simulink model "Projekt_ABS_Sim_Fuzzy"  (R2024b)
settings: Solver=VariableStepAuto  StartTime=0.0  StopTime=10  RelTol=1e-3
values from neighbouring files (symbols this model uses):
  c1 = 0.857    [Projekt_ABS.m]
  c11 = 1.2801    [Projekt_ABS.m]
  c2 = 33.822    [Projekt_ABS.m]
  c22 = 23.99    [Projekt_ABS.m]
  c3 = 0.347    [Projekt_ABS.m]
  c33 = 0.52    [Projekt_ABS.m]
  c4 = 0.035    [Projekt_ABS.m]
  c44 = 0.03    [Projekt_ABS.m]
  g = 9.81    [Projekt_ABS.m]
  J = 1.6    [Projekt_ABS.m]
  m = 1200    [Projekt_ABS.m]
  Mb = 900    [Projekt_ABS.m]
  R = 0.315    [Projekt_ABS.m]
  Ts = 0.01    [Projekt_ABS.m]
  V0 = 40    [Projekt_ABS.m]
undefined symbols (not defined in the file or in its folder): DiscIntNeverNeededParam
libraries: fuzblock x6, simulink x4
settings Model: Creator=abc  LastModifiedBy=abc

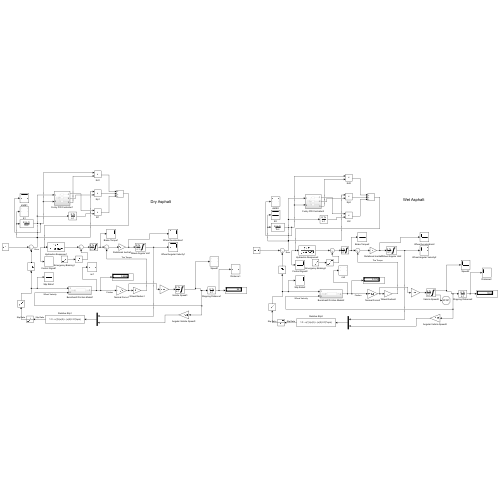
[thumbnail: Simulink's stored preview of the top-level diagram]
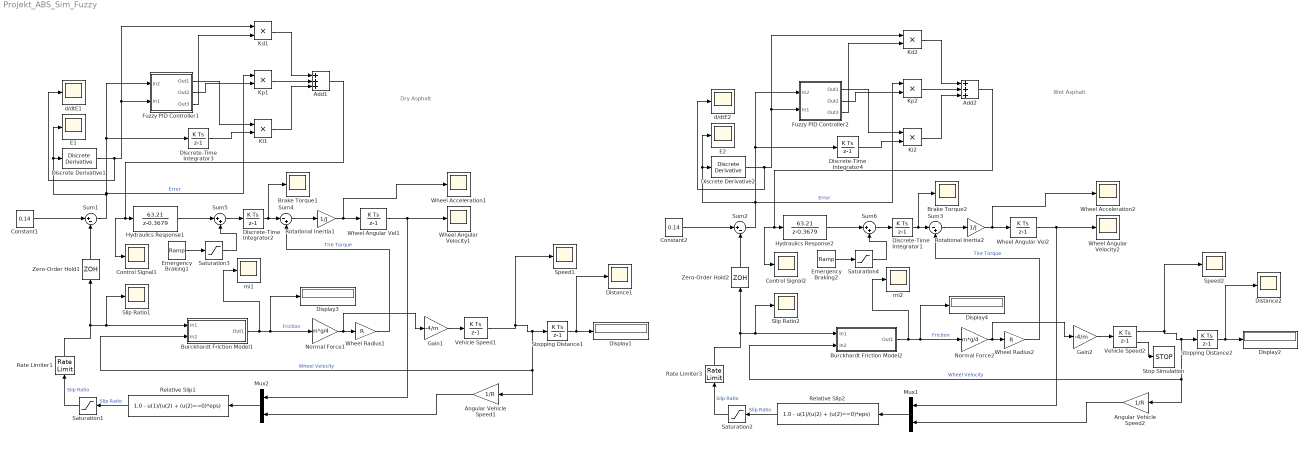
== system Projekt_ABS_Sim_Fuzzy ==
  note: Dry Asphalt
  note: Wet Asphalt
  Add1 : Sum  Inputs=+++
  Add2 : Sum  Inputs=+++
  Angular Vehicle Speed1 : Gain  Gain=1/R
  Angular Vehicle Speed2 : Gain  Gain=1/R
  Brake Torque1 : Scope
  Brake Torque2 : Scope
  Burckhardt Friction Model1 : Subsystem
  Burckhardt Friction Model2 : Subsystem
  Constant1 : Constant  Value=0.14  SampleTime=Ts
  Constant2 : Constant  Value=0.14  SampleTime=Ts
  Control Signal1 : Scope
  Control Signal2 : Scope
  Discrete Derivative1 : simulink/Quick Insert/Discrete/Discrete Derivative  gainval=1.0  ICPrevScaledInput=0.0  OutMin=[]  OutMax=[]  OutDataType=fixdt(1, 16)  OutScaling=2^-10  DoSatur=off
  Discrete Derivative2 : simulink/Quick Insert/Discrete/Discrete Derivative  gainval=1.0  ICPrevScaledInput=0.0  OutMin=[]  OutMax=[]  OutDataType=fixdt(1, 16)  OutScaling=2^-10  DoSatur=off
  Discrete-Time Integrator1 : DiscreteIntegrator  SampleTime=Ts  LimitOutput=on  UpperSaturationLimit=Mb  LowerSaturationLimit=0  ICPrevOutput=DiscIntNeverNeededParam  ICPrevScaledInput=DiscIntNeverNeededParam
  Discrete-Time Integrator2 : DiscreteIntegrator  SampleTime=Ts  LimitOutput=on  UpperSaturationLimit=Mb  LowerSaturationLimit=0  ICPrevOutput=DiscIntNeverNeededParam  ICPrevScaledInput=DiscIntNeverNeededParam
  Discrete-Time Integrator3 : DiscreteIntegrator  SampleTime=Ts  ICPrevOutput=DiscIntNeverNeededParam  ICPrevScaledInput=DiscIntNeverNeededParam
  Discrete-Time Integrator4 : DiscreteIntegrator  SampleTime=Ts  ICPrevOutput=DiscIntNeverNeededParam  ICPrevScaledInput=DiscIntNeverNeededParam
  Display{1..4} (4 alike) : Display
  Distance1 : Scope
  Distance2 : Scope
  E1 : Scope
  E2 : Scope
  Emergency Braking1 : simulink/Sources/Ramp  slope=Mb*2  start=0  InitialOutput=0
  Emergency Braking2 : simulink/Sources/Ramp  slope=Mb*2  start=0  InitialOutput=0
  Fuzzy PID Controller1 : Subsystem
  Fuzzy PID Controller2 : Subsystem
  Gain1 : Gain  Gain=-4/m
  Gain2 : Gain  Gain=-4/m
  Hydraulics Response1 : DiscreteTransferFcn  Numerator=[63.21]  Denominator=[1 -0.3679]  SampleTime=Ts
  Hydraulics Response2 : DiscreteTransferFcn  Numerator=[63.21]  Denominator=[1 -0.3679]  SampleTime=Ts
  Kd1 : Product
  Kd2 : Product
  Ki1 : Product
  Ki2 : Product
  Kp1 : Product
  Kp2 : Product
  Mux1 : Mux  Inputs=2
  Mux2 : Mux  Inputs=2
  Normal Force1 : Gain  Gain=m*g/4
  Normal Force2 : Gain  Gain=m*g/4
  Rate Limiter1 : RateLimiter  RisingSlewLimit=1.5  FallingSlewLimit=-1.5  SampleTimeMode=inherited
  Rate Limiter3 : RateLimiter  RisingSlewLimit=1.5  FallingSlewLimit=-1.5  SampleTimeMode=inherited
  Relative Slip1 : Fcn  Expr=1.0 - u(1)/(u(2) + (u(2)==0)*eps)
  Relative Slip2 : Fcn  Expr=1.0 - u(1)/(u(2) + (u(2)==0)*eps)
  Rotational Inertia1 : Gain  Gain=1/J
  Rotational Inertia2 : Gain  Gain=1/J
  Saturation1 : Saturate  UpperLimit=1  LowerLimit=0
  Saturation2 : Saturate  UpperLimit=1  LowerLimit=0
  Saturation3 : Saturate  UpperLimit=Mb  LowerLimit=0
  Saturation4 : Saturate  UpperLimit=Mb  LowerLimit=0
  Slip Ratio1 : Scope
  Slip Ratio2 : Scope
  Speed1 : Scope
  Speed2 : Scope
  Stop Simulation : Stop
  Stopping Distance1 : DiscreteIntegrator  SampleTime=Ts  ICPrevOutput=DiscIntNeverNeededParam  ICPrevScaledInput=DiscIntNeverNeededParam
  Stopping Distance2 : DiscreteIntegrator  SampleTime=Ts  ICPrevOutput=DiscIntNeverNeededParam  ICPrevScaledInput=DiscIntNeverNeededParam
  Sum1 : Sum  Inputs=|+-
  Sum2 : Sum  Inputs=|+-
  Sum3 : Sum  Inputs=|-+
  Sum4 : Sum  Inputs=|-+
  Sum5 : Sum  Inputs=|++
  Sum6 : Sum  Inputs=|++
  Vehicle Speed1 : DiscreteIntegrator  InitialCondition=V0  SampleTime=Ts  LimitOutput=on  UpperSaturationLimit=1000  LowerSaturationLimit=0  ICPrevOutput=DiscIntNeverNeededParam  ICPrevScaledInput=DiscIntNeverNeededParam
  Vehicle Speed2 : DiscreteIntegrator  InitialCondition=V0  SampleTime=Ts  LimitOutput=on  UpperSaturationLimit=1000  LowerSaturationLimit=0  ShowSaturationPort=on  ICPrevOutput=DiscIntNeverNeededParam  ICPrevScaledInput=DiscIntNeverNeededParam
  Wheel Acceleration1 : Scope
  Wheel Acceleration2 : Scope
  Wheel Angular Vel1 : DiscreteIntegrator  InitialCondition=V0/R  SampleTime=Ts  LimitOutput=on  UpperSaturationLimit=1000  LowerSaturationLimit=0  ICPrevOutput=DiscIntNeverNeededParam  ICPrevScaledInput=DiscIntNeverNeededParam
  Wheel Angular Vel2 : DiscreteIntegrator  InitialCondition=V0/R  SampleTime=Ts  LimitOutput=on  UpperSaturationLimit=1000  LowerSaturationLimit=0  ICPrevOutput=DiscIntNeverNeededParam  ICPrevScaledInput=DiscIntNeverNeededParam
  Wheel Angular Velocity1 : Scope
  Wheel Angular Velocity2 : Scope
  Wheel Radius1 : Gain  Gain=R
  Wheel Radius2 : Gain  Gain=R
  Zero-Order Hold1 : ZeroOrderHold  SampleTime=Ts
  Zero-Order Hold2 : ZeroOrderHold  SampleTime=Ts
  d/dtE1 : Scope
  d/dtE2 : Scope
  mi1 : Scope
  mi2 : Scope
  wires:
  Normal Force1/1 -> Gain1/1, Wheel Radius1/1
  Kp1/1 -> Add1/2
  Sum1/1 -> Kp1/1, Discrete-Time Integrator3/1, Fuzzy PID Controller1/1(In2), Discrete Derivative1/1, E1/1  "Error"
  Zero-Order Hold1/1 -> Sum1/2
  Discrete-Time Integrator2/1 -> Brake Torque1/1, Sum4/1
  Wheel Angular Vel1/1 -> Wheel Angular Velocity1/1, Mux2/1
  Ki1/1 -> Add1/3
  Add1/1 -> Control Signal1/1, Hydraulics Response1/1
  Kd1/1 -> Add1/1
  Discrete Derivative1/1 -> d/dtE1/1, Kd1/1, Fuzzy PID Controller1/2(In1)
  Discrete-Time Integrator3/1 -> Ki1/2
  Fuzzy PID Controller1/1(Out1) -> Ki1/1
  Relative Slip1/1 -> Saturation1/1  "Slip Ratio"
  Saturation1/1 -> Rate Limiter1/1  "Slip Ratio"
  Wheel Radius1/1 -> Sum4/2  "Tire Torque"
  Vehicle Speed1/1 -> Speed1/1, Stopping Distance1/1, Burckhardt Friction Model1/2(In2), Angular Vehicle Speed1/1  "Wheel Velocity"
  Stopping Distance1/1 -> Distance1/1, Display1/1
  Fuzzy PID Controller1/2(Out2) -> Kp1/2
  Burckhardt Friction Model1/1(Out1) -> mi1/1, Display3/1, Normal Force1/1  "Friction"
  Mux2/1 -> Relative Slip1/1
  Rotational Inertia1/1 -> Wheel Angular Vel1/1, Wheel Acceleration1/1
  Rate Limiter1/1 -> Zero-Order Hold1/1, Slip Ratio1/1, Burckhardt Friction Model1/1(In1)
  Gain1/1 -> Vehicle Speed1/1
  Fuzzy PID Controller1/3(Out3) -> Kd1/2
  Sum4/1 -> Rotational Inertia1/1
  Angular Vehicle Speed1/1 -> Mux2/2
  Constant1/1 -> Sum1/1
  Emergency Braking1/1 -> Saturation3/1
  Saturation3/1 -> Sum5/2
  Hydraulics Response1/1 -> Sum5/1
  Sum5/1 -> Discrete-Time Integrator2/1
  Discrete Derivative2/1 -> d/dtE2/1, Kd2/1, Fuzzy PID Controller2/2(In1)
  Gain2/1 -> Vehicle Speed2/1
  Kd2/1 -> Add2/1
  Vehicle Speed2/1 -> Stopping Distance2/1, Burckhardt Friction Model2/2(In2), Angular Vehicle Speed2/1, Speed2/1  "Wheel Velocity"
  Ki2/1 -> Add2/3
  Hydraulics Response2/1 -> Sum6/1
  Wheel Angular Vel2/1 -> Wheel Angular Velocity2/1, Mux1/1
  Fuzzy PID Controller2/1(Out1) -> Ki2/1
  Saturation2/1 -> Rate Limiter3/1  "Slip Ratio"
  Rate Limiter3/1 -> Zero-Order Hold2/1, Slip Ratio2/1, Burckhardt Friction Model2/1(In1)
  Kp2/1 -> Add2/2
  Normal Force2/1 -> Gain2/1, Wheel Radius2/1
  Emergency Braking2/1 -> Saturation4/1
  Zero-Order Hold2/1 -> Sum2/2
  Burckhardt Friction Model2/1(Out1) -> mi2/1, Display4/1, Normal Force2/1  "Friction"
  Mux1/1 -> Relative Slip2/1
  Saturation4/1 -> Sum6/2
  Fuzzy PID Controller2/2(Out2) -> Kp2/2
  Sum3/1 -> Rotational Inertia2/1
  Wheel Radius2/1 -> Sum3/2  "Tire Torque"
  Sum2/1 -> Kp2/1, Discrete-Time Integrator4/1, Fuzzy PID Controller2/1(In2), Discrete Derivative2/1, E2/1  "Error"
  Sum6/1 -> Discrete-Time Integrator1/1
  Stopping Distance2/1 -> Distance2/1, Display2/1
  Angular Vehicle Speed2/1 -> Mux1/2
  Relative Slip2/1 -> Saturation2/1  "Slip Ratio"
  Discrete-Time Integrator1/1 -> Brake Torque2/1, Sum3/1
  Fuzzy PID Controller2/3(Out3) -> Kd2/2
  Discrete-Time Integrator4/1 -> Ki2/2
  Constant2/1 -> Sum2/1
  Add2/1 -> Control Signal2/1, Hydraulics Response2/1
  Rotational Inertia2/1 -> Wheel Angular Vel2/1, Wheel Acceleration2/1
  Vehicle Speed2/2 -> Stop Simulation/1

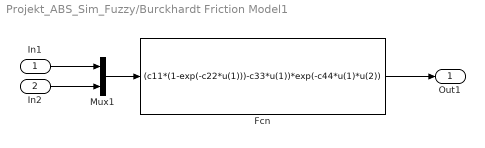
== system Projekt_ABS_Sim_Fuzzy/Burckhardt Friction Model1 ==
  In1 : Inport
  In2 : Inport  Port=2
  Fcn : Fcn  Expr=(c11*(1-exp(-c22*u(1)))-c33*u(1))*exp(-c44*u(1)*u(2))
  Mux1 : Mux  Inputs=2
  Out1 : Outport
  wires:
  In2/1 -> Mux1/2
  Mux1/1 -> Fcn/1
  In1/1 -> Mux1/1
  Fcn/1 -> Out1/1

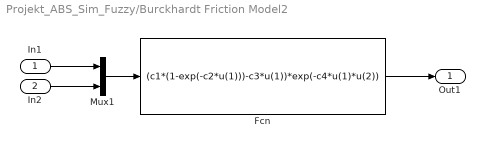
== system Projekt_ABS_Sim_Fuzzy/Burckhardt Friction Model2 ==
  In1 : Inport
  In2 : Inport  Port=2
  Fcn : Fcn  Expr=(c1*(1-exp(-c2*u(1)))-c3*u(1))*exp(-c4*u(1)*u(2))
  Mux1 : Mux  Inputs=2
  Out1 : Outport
  wires:
  In2/1 -> Mux1/2
  Mux1/1 -> Fcn/1
  In1/1 -> Mux1/1
  Fcn/1 -> Out1/1

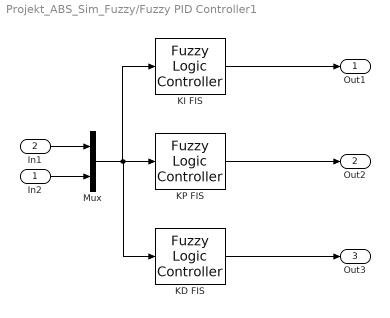
== system Projekt_ABS_Sim_Fuzzy/Fuzzy PID Controller1 ==
  In2 : Inport
  In1 : Inport  Port=2
  KD FIS : fuzblock/Fuzzy Logic  Controller  FIS='KD.fis'  OutputSampleNumber=101  DataType=double  FuzzifiedInputs=off  RuleFiringStrengths=off  RuleOutputs=off  AggregatedOutputs=off  SimulateUsing=Interpreted execution  OutOfRangeInputValueMessage=warning  NoRuleFiredMessage=warning  EmptyOutputFuzzySetMessage=warning
  KI FIS : fuzblock/Fuzzy Logic  Controller  FIS='KI.fis'  OutputSampleNumber=101  DataType=double  FuzzifiedInputs=off  RuleFiringStrengths=off  RuleOutputs=off  AggregatedOutputs=off  SimulateUsing=Interpreted execution  OutOfRangeInputValueMessage=warning  NoRuleFiredMessage=warning  EmptyOutputFuzzySetMessage=warning
  KP FIS : fuzblock/Fuzzy Logic  Controller  FIS='KP.fis'  OutputSampleNumber=101  DataType=double  FuzzifiedInputs=off  RuleFiringStrengths=off  RuleOutputs=off  AggregatedOutputs=off  SimulateUsing=Interpreted execution  OutOfRangeInputValueMessage=warning  NoRuleFiredMessage=warning  EmptyOutputFuzzySetMessage=warning
  Mux : Mux  Inputs=2
  Out1 : Outport
  Out2 : Outport  Port=2
  Out3 : Outport  Port=3
  wires:
  Mux/1 -> KI FIS/1, KD FIS/1, KP FIS/1
  In1/1 -> Mux/1
  KI FIS/1 -> Out1/1
  KD FIS/1 -> Out3/1
  KP FIS/1 -> Out2/1
  In2/1 -> Mux/2

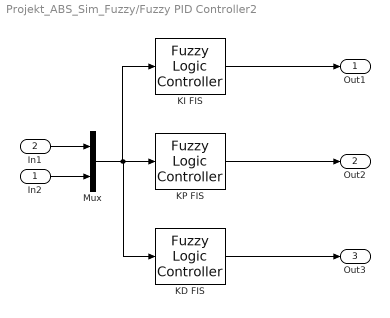
== system Projekt_ABS_Sim_Fuzzy/Fuzzy PID Controller2 ==
  In2 : Inport
  In1 : Inport  Port=2
  KD FIS : fuzblock/Fuzzy Logic  Controller  FIS='KD.fis'  OutputSampleNumber=101  DataType=double  FuzzifiedInputs=off  RuleFiringStrengths=off  RuleOutputs=off  AggregatedOutputs=off  SimulateUsing=Interpreted execution  OutOfRangeInputValueMessage=warning  NoRuleFiredMessage=warning  EmptyOutputFuzzySetMessage=warning
  KI FIS : fuzblock/Fuzzy Logic  Controller  FIS='KI.fis'  OutputSampleNumber=101  DataType=double  FuzzifiedInputs=off  RuleFiringStrengths=off  RuleOutputs=off  AggregatedOutputs=off  SimulateUsing=Interpreted execution  OutOfRangeInputValueMessage=warning  NoRuleFiredMessage=warning  EmptyOutputFuzzySetMessage=warning
  KP FIS : fuzblock/Fuzzy Logic  Controller  FIS='KP.fis'  OutputSampleNumber=101  DataType=double  FuzzifiedInputs=off  RuleFiringStrengths=off  RuleOutputs=off  AggregatedOutputs=off  SimulateUsing=Interpreted execution  OutOfRangeInputValueMessage=warning  NoRuleFiredMessage=warning  EmptyOutputFuzzySetMessage=warning
  Mux : Mux  Inputs=2
  Out1 : Outport
  Out2 : Outport  Port=2
  Out3 : Outport  Port=3
  wires:
  Mux/1 -> KI FIS/1, KD FIS/1, KP FIS/1
  In1/1 -> Mux/1
  KI FIS/1 -> Out1/1
  KD FIS/1 -> Out3/1
  KP FIS/1 -> Out2/1
  In2/1 -> Mux/2
